simulink model "robusnost_sim"  (R2020a)
settings: Solver=VariableStepAuto  StartTime=0.0  StopTime=10.0  RelTol=1e-3
values from neighbouring files (symbols this model uses):
  C = 470e-6    (= 0.00047)    [linearizacija_simbolicki_script.m]    (also in linearizacija_simbolicki_skripta.m)
  E = 12    [linearizacija_simbolicki_script.m]    (also in linearizacija_simbolicki_skripta.m)
  L = 15.91e-3    (= 0.01591)    [linearizacija_simbolicki_script.m]    (also in linearizacija_simbolicki_skripta.m)
  R = 52    [linearizacija_simbolicki_script.m]    (also in linearizacija_simbolicki_skripta.m)
  ue = eval(ue)    [linearizacija_simbolicki_script.m]    (also in linearizacija_simbolicki_skripta.m)
  x2e = -22.5    [linearizacija_simbolicki_script.m]    (also in linearizacija_simbolicki_skripta.m)
settings Model: Creator=H-BRIDGES  LastModifiedBy=H-BRIDGES

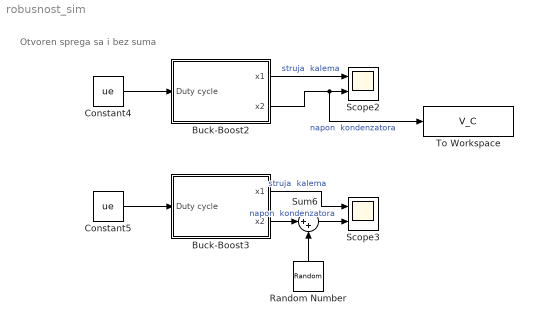
== system robusnost_sim ==
  note: Otvoren sprega sa i bez suma
  Buck-Boost2 : Subsystem
  Buck-Boost3 : Subsystem
  Constant4 : Constant  Value=ue
  Constant5 : Constant  Value=ue
  Random Number : RandomNumber  Variance=(0.05 * abs(x2e))^2  SampleTime=1e-3
  Scope2 : Scope  NumInputPorts=2
  Scope3 : Scope  NumInputPorts=2
  Sum6 : Sum  Inputs=|++
  To Workspace : ToWorkspace  VariableName=V_C  SaveFormat=Timeseries  SampleTime=-1
  wires:
  Buck-Boost2/2(x2) -> To Workspace/1, Scope2/2  "napon  kondenzatora"
  Buck-Boost3/2(x2) -> Sum6/1  "napon  kondenzatora"
  Random Number/1 -> Sum6/2
  Constant4/1 -> Buck-Boost2/1(Duty cycle)
  Sum6/1 -> Scope3/2
  Buck-Boost3/1(x1) -> Scope3/1  "struja  kalema"
  Buck-Boost2/1(x1) -> Scope2/1  "struja  kalema"
  Constant5/1 -> Buck-Boost3/1(Duty cycle)

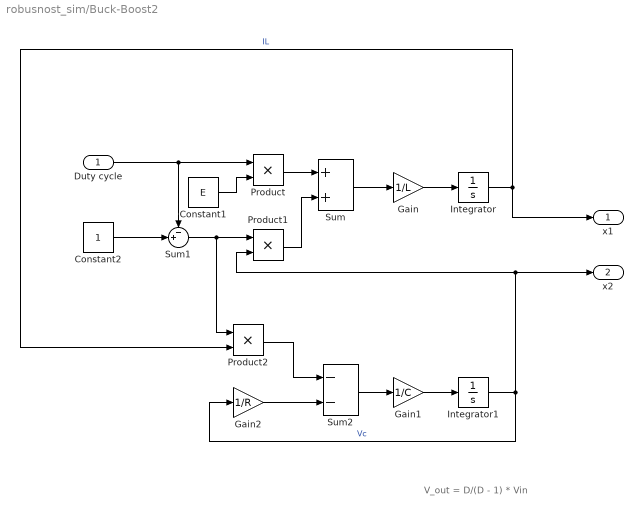
== system robusnost_sim/Buck-Boost2 ==
  note: V_out = D/(D - 1) * Vin
  Duty cycle : Inport
  Constant1 : Constant  Value=E
  Constant2 : Constant
  Gain : Gain  Gain=1/L
  Gain1 : Gain  Gain=1/C
  Gain2 : Gain  Gain=1/R
  Integrator : Integrator
  Integrator1 : Integrator
  Product : Product
  Product1 : Product
  Product2 : Product
  Sum : Sum
  Sum1 : Sum  Inputs=-+|
  Sum2 : Sum  Inputs=--
  x1 : Outport
  x2 : Outport  Port=2
  wires:
  Product/1 -> Sum/1
  Product1/1 -> Sum/2
  Sum2/1 -> Gain1/1
  Constant1/1 -> Product/2
  Integrator1/1 -> Gain2/1, x2/1, Product1/2  "Vc"
  Gain1/1 -> Integrator1/1
  Constant2/1 -> Sum1/2
  Integrator/1 -> x1/1, Product2/2  "IL"
  Sum/1 -> Gain/1
  Gain2/1 -> Sum2/2
  Sum1/1 -> Product2/1, Product1/1
  Duty cycle/1 -> Sum1/1, Product/1
  Product2/1 -> Sum2/1
  Gain/1 -> Integrator/1

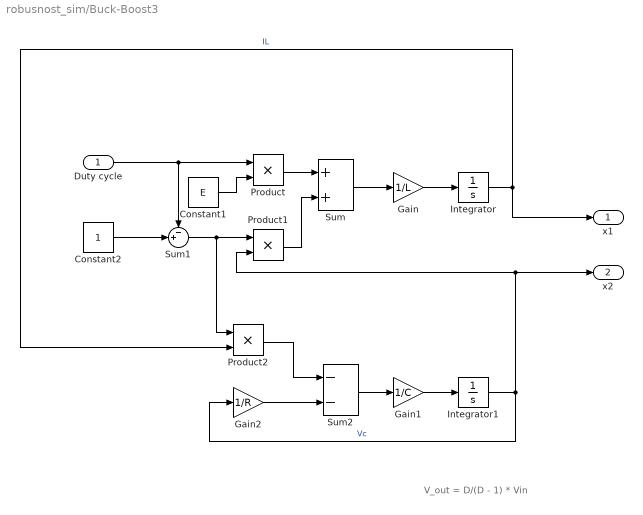
== system robusnost_sim/Buck-Boost3 ==
  note: V_out = D/(D - 1) * Vin
  Duty cycle : Inport
  Constant1 : Constant  Value=E
  Constant2 : Constant
  Gain : Gain  Gain=1/L
  Gain1 : Gain  Gain=1/C
  Gain2 : Gain  Gain=1/R
  Integrator : Integrator
  Integrator1 : Integrator
  Product : Product
  Product1 : Product
  Product2 : Product
  Sum : Sum
  Sum1 : Sum  Inputs=-+|
  Sum2 : Sum  Inputs=--
  x1 : Outport
  x2 : Outport  Port=2
  wires:
  Product/1 -> Sum/1
  Product1/1 -> Sum/2
  Sum2/1 -> Gain1/1
  Constant1/1 -> Product/2
  Integrator1/1 -> Gain2/1, x2/1, Product1/2  "Vc"
  Gain1/1 -> Integrator1/1
  Constant2/1 -> Sum1/2
  Integrator/1 -> x1/1, Product2/2  "IL"
  Sum/1 -> Gain/1
  Gain2/1 -> Sum2/2
  Sum1/1 -> Product2/1, Product1/1
  Duty cycle/1 -> Sum1/1, Product/1
  Product2/1 -> Sum2/1
  Gain/1 -> Integrator/1
